simulink model "Sum1"  (R2020b)
settings: Solver=VariableStepAuto  StartTime=0.0  StopTime=10.0  RelTol=1e-3
undefined symbols (not defined in the file): b, k1, k12, m1, m2
settings Model: Creator=Aradhana desai  LastModifiedBy=Aradhana desai

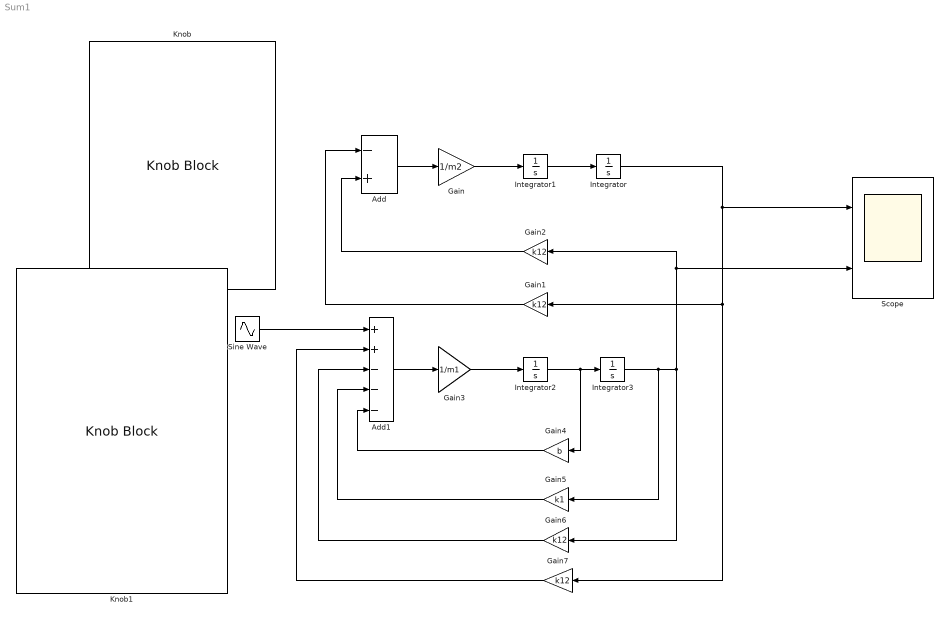
== system Sum1 ==
  Add : Sum  Inputs=-+
  Add1 : Sum  Inputs=++---
  Gain : Gain  Gain=1/m2
  Gain{1..2,6..7} (4 alike) : Gain  Gain=k12
  Gain3 : Gain  Gain=1/m1
  Gain4 : Gain  Gain=b
  Gain5 : Gain  Gain=k1
  Integrator{,1..3} (4 alike) : Integrator
  Knob : KnobBlock
  Knob1 : KnobBlock  ScaleMin=-500  ScaleMax=10000
  Scope : Scope  NumInputPorts=2
  Sine Wave : Sin  SampleTime=0
  wires:
  Integrator2/1 -> Gain4/1, Integrator3/1
  Gain3/1 -> Integrator2/1
  Add1/1 -> Gain3/1
  Gain4/1 -> Add1/5
  Gain5/1 -> Add1/4
  Gain6/1 -> Add1/3
  Gain7/1 -> Add1/2
  Sine Wave/1 -> Add1/1
  Add/1 -> Gain/1
  Gain/1 -> Integrator1/1
  Integrator1/1 -> Integrator/1
  Integrator/1 -> Gain1/1, Gain7/1, Scope/1
  Gain1/1 -> Add/1
  Gain2/1 -> Add/2
  Integrator3/1 -> Gain5/1, Gain2/1, Scope/2, Gain6/1
